simulink model "lab4_2"  (R2021a)
settings: Solver=VariableStepAuto  StartTime=0.0  StopTime=20.0  RelTol=1e-10  AbsTol=1e-10
values from neighbouring files (symbols this model uses):
  d_bar = (Ra/Kt) * tau_l    (= 3)    [lab4.m]
  Kaw = 1/Ti    [lab4.m]
  thetades = pi/2    (= 1.57079632679)    [lab4.m]
  Ti = 1/(omega_bar/10)    [lab4.m]
  Vlim = 5    [lab4.m]
libraries: cstblocks x2
settings Model: Creator=markalex  LastModifiedBy=markalex

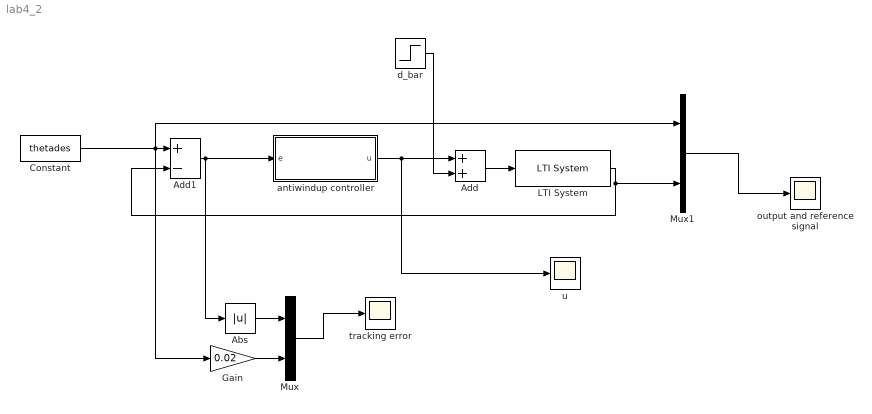
== system lab4_2 ==
  Abs : Abs
  Add : Sum
  Add1 : Sum  Inputs=+-
  Constant : Constant  Value=thetades
  Gain : Gain  Gain=0.02
  LTI System : cstblocks/LTI System  sys=G  IC=[]
  Mux : Mux  Inputs=2
  Mux1 : Mux  Inputs=2
  antiwindup controller : Subsystem
  d_bar : Step  Time=5  After=d_bar  SampleTime=0
  output and reference signal : Scope
  tracking error : Scope
  u : Scope
  wires:
  Mux1/1 -> output and reference signal/1
  Mux/1 -> tracking error/1
  Constant/1 -> Mux1/1, Add1/1, Gain/1
  Add1/1 -> antiwindup controller/1(e), Abs/1
  Add/1 -> LTI System/1
  LTI System/1 -> Add1/2, Mux1/2
  d_bar/1 -> Add/2
  Gain/1 -> Mux/2
  Abs/1 -> Mux/1
  antiwindup controller/1(u) -> Add/1, u/1

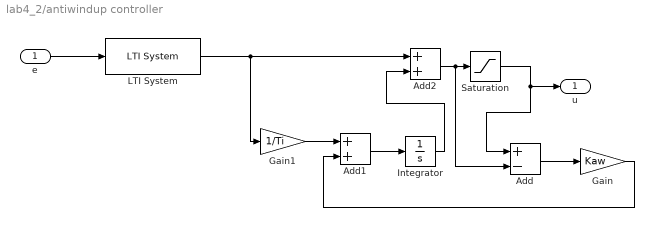
== system lab4_2/antiwindup controller ==
  e : Inport
  Add : Sum  Inputs=+-
  Add1 : Sum
  Add2 : Sum
  Gain : Gain  Gain=Kaw
  Gain1 : Gain  Gain=1/Ti
  Integrator : Integrator
  LTI System : cstblocks/LTI System  sys=C1  IC=[]
  Saturation : Saturate  UpperLimit=Vlim  LowerLimit=-Vlim
  u : Outport
  wires:
  e/1 -> LTI System/1
  LTI System/1 -> Gain1/1, Add2/1
  Add2/1 -> Add/2, Saturation/1
  Saturation/1 -> Add/1, u/1
  Gain1/1 -> Add1/1
  Add1/1 -> Integrator/1
  Integrator/1 -> Add2/2
  Add/1 -> Gain/1
  Gain/1 -> Add1/2
